simulink model "simulasEX1"  (R2024a)
settings: Solver=VariableStepAuto  StartTime=0.0  StopTime=1  FixedStep=0.0000001  RelTol=1e-3
undefined symbols (not defined in the file): K, T
settings Model: Creator=a2408732  LastModifiedBy=a2408732

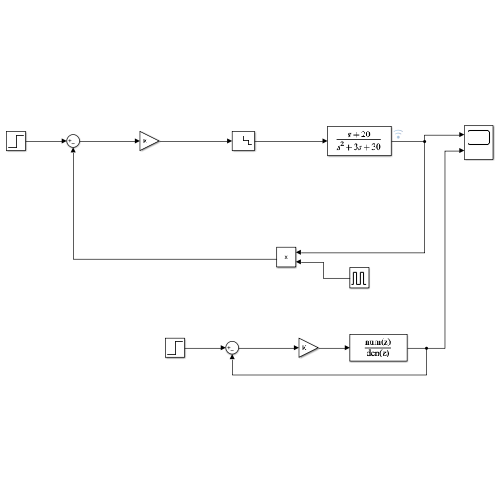
[thumbnail: Simulink's stored preview of the top-level diagram]
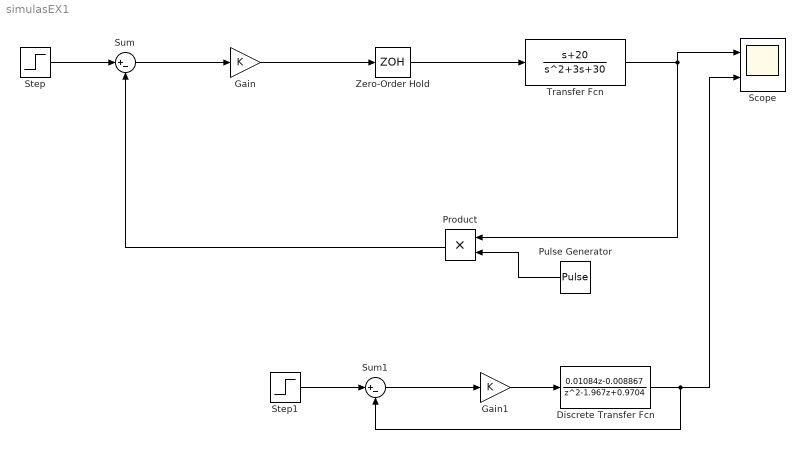
== system simulasEX1 ==
  Discrete Transfer Fcn : DiscreteTransferFcn  Numerator=[0.01084 -0.008867]  Denominator=[1 -1.967 0.9704]
  Gain : Gain  Gain=K
  Gain1 : Gain  Gain=K
  Product : Product
  Pulse Generator : DiscretePulseGenerator  PulseType=Time based  Period=T  PulseWidth=0.1
  Scope : Scope  NumInputPorts=2
  Step : Step  Time=0  SampleTime=0
  Step1 : Step  Time=0  SampleTime=0
  Sum : Sum  Inputs=|+-
  Sum1 : Sum  Inputs=|+-
  Transfer Fcn : TransferFcn  Numerator=[1 20]  Denominator=[1 3 30]
  Zero-Order Hold : ZeroOrderHold  SampleTime=T
  wires:
  Transfer Fcn/1 -> Product/1, Scope/1
  Pulse Generator/1 -> Product/2
  Zero-Order Hold/1 -> Transfer Fcn/1
  Gain/1 -> Zero-Order Hold/1
  Sum/1 -> Gain/1
  Step/1 -> Sum/1
  Product/1 -> Sum/2
  Sum1/1 -> Gain1/1
  Step1/1 -> Sum1/1
  Gain1/1 -> Discrete Transfer Fcn/1
  Discrete Transfer Fcn/1 -> Sum1/2, Scope/2
